simulink model "lab5"  (R2015a)
settings: Solver=ode45  StartTime=0.0  StopTime=500.0  MaxStep=0.2  RelTol=1e-3
values from neighbouring files (symbols this model uses):
  ddMax = 3    [lab5go.m]    (also in sysdat.m)
  deltaMax = 30    [lab5go.m]    (also in sysdat.m)
  fConst = 0    [lab5go.m]    (also in sysdat.m)
  K = 0.08    [lab5go.m]    (also in sysdat.m)
  Kc = 1.04    [lab5go.m]    (also in sysdat.m)
  phiZad = 30    [lab5go.m]    (also in sysdat.m)
  Ti = 200    [lab5go.m]    (also in sysdat.m)
  Tr = 1    [lab5go.m]    (also in sysdat.m)
  Ts = 16.4    [lab5go.m]    (also in sysdat.m)
  Ts0 = Ts    (= 16.4)    [lab5go.m]
settings Model: Creator=vbox  LastModifiedBy=vbox
settings DataIOCC: InspectSignalLogs=on

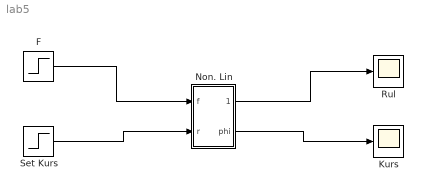
== system lab5 ==
  F : Step  After=fConst  SampleTime=0
  Kurs : Scope
      settings: SaveName=phi
  Non. Lin : Subsystem
  Rul : Scope
      settings: TimeRange=100  YMin=0  YMax=400  SaveName=delta
  Set Kurs : Step  Time=0  After=phiZad  SampleTime=0
  wires:
  Non. Lin/2(phi) -> Kurs/1
  Set Kurs/1 -> Non. Lin/2(r)
  F/1 -> Non. Lin/1(f)
  Non. Lin/1(delta) -> Rul/1

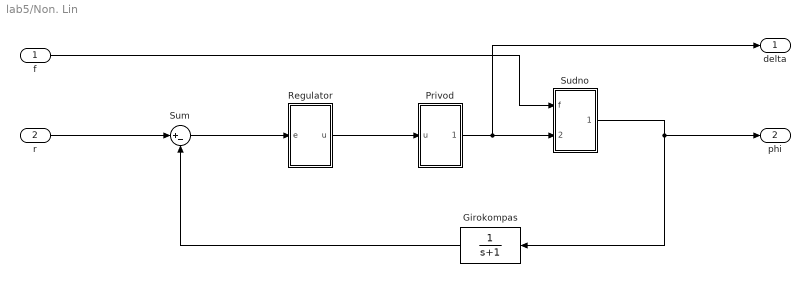
== system lab5/Non. Lin ==
  f : Inport
  r : Inport  Port=2
  Girokompas : TransferFcn  Denominator=[1 1]
  Privod : Subsystem
  Regulator : Subsystem
  Sudno : Subsystem
  Sum : Sum  Inputs=|+-
  delta : Outport
  phi : Outport  Port=2
  wires:
  Girokompas/1 -> Sum/2
  r/1 -> Sum/1
  Sudno/1(phi) -> phi/1, Girokompas/1
  Sum/1 -> Regulator/1(e)
  f/1 -> Sudno/1(f)
  Privod/1(delta) -> delta/1, Sudno/2(delta)
  Regulator/1(u) -> Privod/1(u)

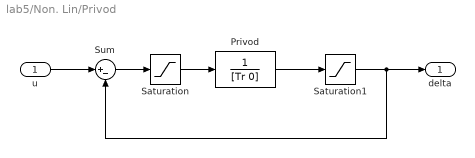
== system lab5/Non. Lin/Privod ==
  u : Inport
  Privod : TransferFcn  Denominator=[Tr 0]
  Saturation : Saturate  UpperLimit=Tr*ddMax  LowerLimit=-Tr*ddMax
      settings: LockScale=on
  Saturation1 : Saturate  UpperLimit=deltaMax  LowerLimit=-deltaMax
  Sum : Sum  Inputs=|+-
  delta : Outport
  wires:
  u/1 -> Sum/1
  Sum/1 -> Saturation/1
  Saturation/1 -> Privod/1
  Privod/1 -> Saturation1/1
  Saturation1/1 -> Sum/2, delta/1

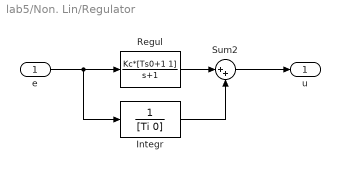
== system lab5/Non. Lin/Regulator ==
  e : Inport
  Integr : TransferFcn  Denominator=[Ti 0]
  Regul : TransferFcn  Numerator=Kc*[Ts0+1 1]  Denominator=[1 1]
  Sum2 : Sum  Inputs=|++
  u : Outport
  wires:
  e/1 -> Integr/1, Regul/1
  Sum2/1 -> u/1
  Regul/1 -> Sum2/1
  Integr/1 -> Sum2/2

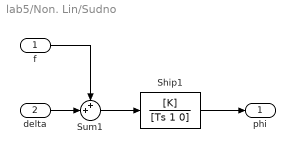
== system lab5/Non. Lin/Sudno ==
  f : Inport
  delta : Inport  Port=2
  Ship1 : TransferFcn  Numerator=[K]  Denominator=[Ts 1 0]
  Sum1 : Sum  Inputs=++|
  phi : Outport
  wires:
  Sum1/1 -> Ship1/1
  Ship1/1 -> phi/1
  f/1 -> Sum1/1
  delta/1 -> Sum1/2
